simulink model "fsm_implemented"  (R2022b)
settings: Solver=VariableStepAuto  StartTime=0.0  StopTime=T  MaxStep=MaxStep  RelTol=RelTol
values from neighbouring files (symbols this model uses):
  J = 20    [initialization.m]
  T = 10    [initialization.m]
libraries: HyEQ_Library x2
settings Model: Creator=tom  LastModifiedBy=tom

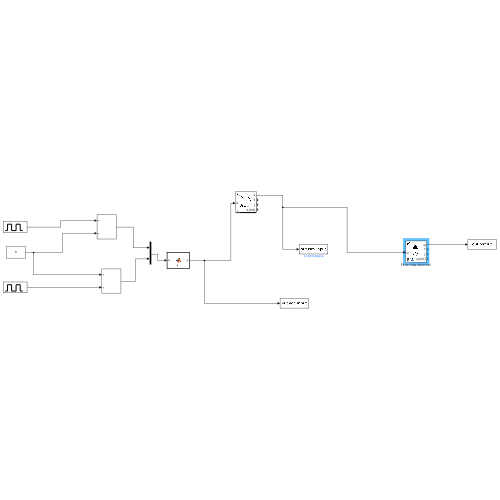
[thumbnail: Simulink's stored preview of the top-level diagram]
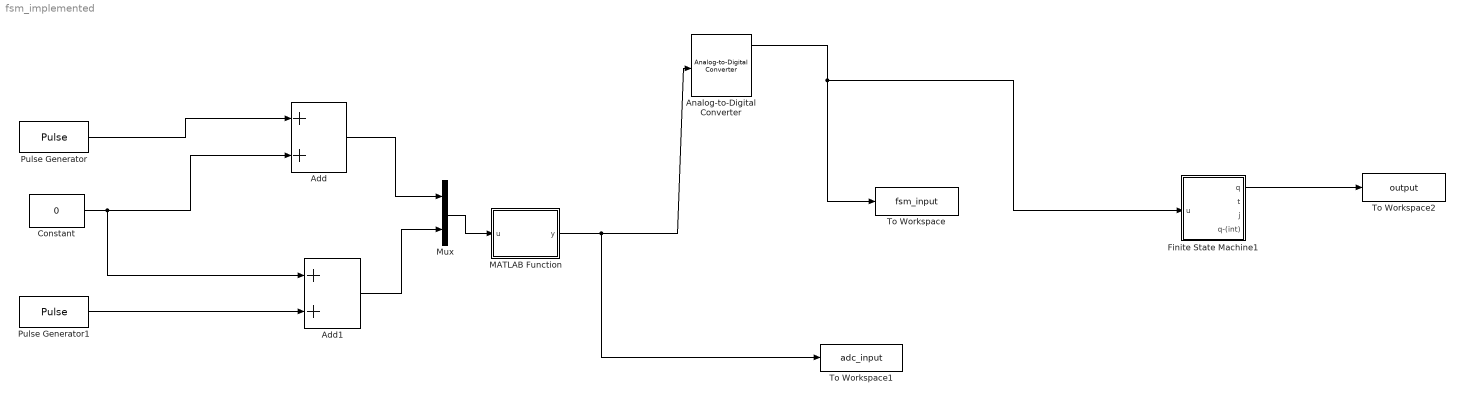
== system fsm_implemented ==
  Add : Sum
  Add1 : Sum
  Analog-to-Digital Converter : HyEQ_Library/Cyber Physical Systems/Analog-to-Digital Converter  sample_time=1  u0=[0]  tau0=0  T=T  J=J
      settings: SourceProductName=Hybrid Equations Toolbox
  Constant : Constant  Value=0
  Finite State Machine1 : Subsystem  LoadFcn=set_param(gcb,'LinkStatus','none')  mask(Finite State Machine (FSM)){q0=0, input_dim=2, T=T, J=J}
      mask prompts: q0 "Initial state (column vector)"; input_dim "Input dimension (nonnegative integer)"; T "Flow Horizon (nonnegative real)"; J "Jump Horizon (nonnegative integer)"
      mask help:
      | To define the FSM:
      | 1. Select the block,
      | 2. "Look inside" the block: Either open the context menu and select Mask > Look Under Mask, or click the arrow in the bottom-left corner of the block.
      | 3. Edit the flow set C, jump set D, and jump map g.
      mask init:
      | state_dim = numel(q0);
      settings: CopyFcn=|
      | set_param(gcb,'LinkStatus','none'),
      | set_param(gcs, 'MaxStep', 'MaxStep', 'RelTol', 'RelTol','StopTime', 'T')
      mask Help: eval hybrid.internal.openHelp('CPS_finite_state_machine')
      mask TypeOptions T: Integrator System/T
      mask TypeOptions J: Integrator System/J
      mask DialogControl Control2 Prompt: CPS Components Documentation
      mask DialogControl Control2 Callback: hybrid.internal.openHelp('CPS_Components')
      mask DialogControl Container4 Prompt: Configuration
      mask Display:
      | image('FSM.jpg')
      | port_label('output', 1, 'q')
      | port_label('output', 2, 't')
      | port_label('output', 3, 'j')
      | port_label('output', 4, 'q-(int)')
      | port_label('input', 1, 'u')
  MATLAB Function : MATLAB Function  TreatAsAtomicUnit=on
  Mux : Mux  Inputs=2
  Pulse Generator : DiscretePulseGenerator  PulseType=Time based  Period=10  PulseWidth=5
  Pulse Generator1 : DiscretePulseGenerator  PulseType=Time based  Period=10  PulseWidth=5
  To Workspace : ToWorkspace  VariableName=fsm_input  SaveFormat=Timeseries  SampleTime=-1
  To Workspace1 : ToWorkspace  VariableName=adc_input  SaveFormat=Timeseries  SampleTime=-1
  To Workspace2 : ToWorkspace  VariableName=output  SaveFormat=Timeseries  SampleTime=-1
  wires:
  Pulse Generator/1 -> Add/1
  Pulse Generator1/1 -> Add1/2
  Constant/1 -> Add1/1, Add/2
  Add/1 -> Mux/1
  Add1/1 -> Mux/2
  MATLAB Function/1(y) -> To Workspace1/1, Analog-to-Digital Converter/1
  Mux/1 -> MATLAB Function/1(u)
  Analog-to-Digital Converter/1 -> Finite State Machine1/1(u), To Workspace/1
  Finite State Machine1/1(q) -> To Workspace2/1

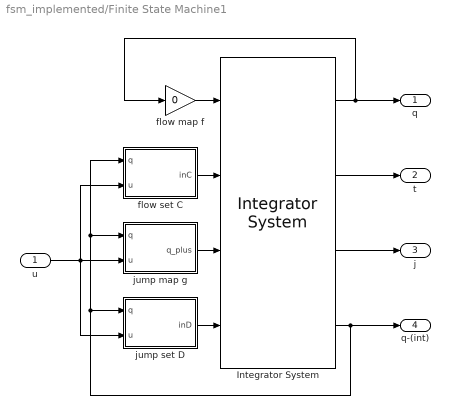
== system fsm_implemented/Finite State Machine1 ==
  u : Inport  PortDimensions=input_dim
  Integrator System : HyEQ_Library/Other/Integrator System  Priority=2  T=T  J=J  x0=q0  rule=1
      settings: SourceProductName=Hybrid Equations Toolbox
  flow map f : Gain  Gain=0
  flow set C : MATLAB Function  TreatAsAtomicUnit=on
  jump map g : MATLAB Function  TreatAsAtomicUnit=on
  jump set D : MATLAB Function  TreatAsAtomicUnit=on
  q : Outport  PortDimensions=state_dim
  t : Outport  Port=2  PortDimensions=1
  j : Outport  Port=3  PortDimensions=1
  q-(int) : Outport  Port=4  PortDimensions=state_dim
  wires:
  jump map g/1(q_plus) -> Integrator System/3
  jump set D/1(inD) -> Integrator System/4
  u/1 -> jump map g/2(u), jump set D/2(u), flow set C/2(u)
  Integrator System/3 -> j/1
  Integrator System/2 -> t/1
  flow set C/1(inC) -> Integrator System/2
  Integrator System/1 -> q/1, flow map f/1
  Integrator System/4 -> q-(int)/1, flow set C/1(q), jump map g/1(q), jump set D/1(q)
  flow map f/1 -> Integrator System/1

== matlab function fsm_implemented/MATLAB Function ==
  data: u input; y output
function y = fcn(u)

y = 1-u(1);

== matlab function fsm_implemented/Finite State Machine1/jump map g ==
  data: q input size=state_dim; u input size=input_dim; q_plus output size=state_dim
function q_plus = g(q, u)
    % Jump map for finite state machine.
    % u has 2 dimensions, input (m_s (u(1))) and time (u(2))
    if (u(1) == 0) && ((q == 1) || (q == 2))
        qplus = 1;       
    elseif (u(1) == 0) && (q == 3)
        qplus = q;
    elseif (u(1) == 1) && (q == 1)
        qplus = 2;
    elseif (u(1) == 1) && ((q == 2) || (q == 3))
        qplus = 3;   
    else
        qplus = q;  % this line is not in original program and is added to fix 'if' syntax error
    end
    q_plus = qplus;
end

== matlab function fsm_implemented/Finite State Machine1/jump set D ==
  data: q input size=state_dim; u input size=input_dim; inD output size=1
function inD  = D(q, u) 
    % Jump set indicator finite state machine.

    % Specify conditions for when the system should jump.
    inD = any(u ~= q); 
end

== matlab function fsm_implemented/Finite State Machine1/flow set C ==
  data: q input size=state_dim; u input size=input_dim; inC output size=1
function inC  = C(q, u) 
    % Flow set indicator function for finite state machine.
    
    % Specify conditions for when the system should flow.
    %inC = all(u == q);
    inC = 1;
end
